simulink model "example_of_spead_control"  (R2021a)
settings: Solver=VariableStepAuto  StartTime=0.0  StopTime=10.0  RelTol=1e-3
libraries: simulink x1
settings Model: Creator=YasserNet  LastModifiedBy=YasserNet

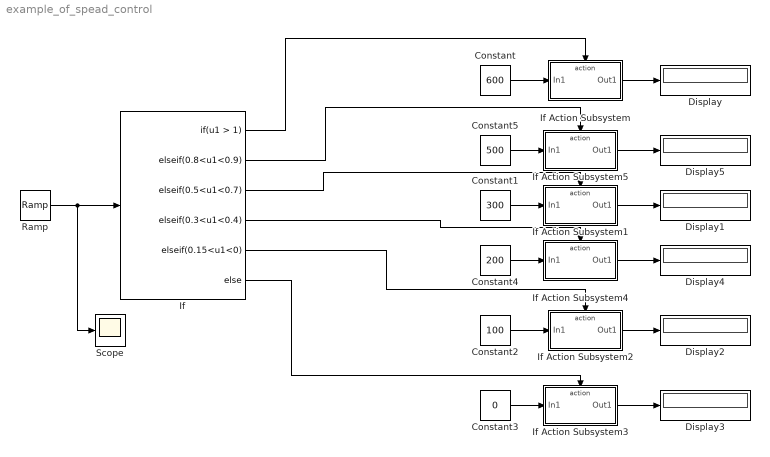
== system example_of_spead_control ==
  Constant : Constant  Value=600
  Constant1 : Constant  Value=300
  Constant2 : Constant  Value=100
  Constant3 : Constant  Value=0
  Constant4 : Constant  Value=200
  Constant5 : Constant  Value=500
  Display{,1..5} (6 alike) : Display
  If : If  IfExpression=u1 > 1  ElseIfExpressions=0.8<u1<0.9,0.5<u1<0.7,0.3<u1<0.4,0.15<u1<0
  If Action Subsystem : Subsystem  TreatAsAtomicUnit=on
  If Action Subsystem1 : Subsystem  TreatAsAtomicUnit=on
  If Action Subsystem2 : Subsystem  TreatAsAtomicUnit=on
  If Action Subsystem3 : Subsystem  TreatAsAtomicUnit=on
  If Action Subsystem4 : Subsystem  TreatAsAtomicUnit=on
  If Action Subsystem5 : Subsystem  TreatAsAtomicUnit=on
  Ramp : simulink/Sources/Ramp  slope=1  start=1  InitialOutput=6
  Scope : Scope
  wires:
  Ramp/1 -> Scope/1, If/1
  If Action Subsystem/1(Out1) -> Display/1
  Constant/1 -> If Action Subsystem/1(In1)
  Constant1/1 -> If Action Subsystem1/1(In1)
  If Action Subsystem1/1(Out1) -> Display1/1
  If Action Subsystem2/1(Out1) -> Display2/1
  Constant2/1 -> If Action Subsystem2/1(In1)
  Constant3/1 -> If Action Subsystem3/1(In1)
  If Action Subsystem3/1(Out1) -> Display3/1
  If Action Subsystem4/1(Out1) -> Display4/1
  Constant4/1 -> If Action Subsystem4/1(In1)
  Constant5/1 -> If Action Subsystem5/1(In1)
  If Action Subsystem5/1(Out1) -> Display5/1
  If/1 -> If Action Subsystem/Action
  If/2 -> If Action Subsystem5/Action
  If/6 -> If Action Subsystem3/Action
  If/3 -> If Action Subsystem1/Action
  If/4 -> If Action Subsystem4/Action
  If/5 -> If Action Subsystem2/Action

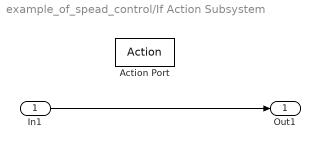
== system example_of_spead_control/If Action Subsystem ==
  In1 : Inport
  Action Port : ActionPort  ActionPortLabel=if(u1 > 1)
  Out1 : Outport
  wires:
  In1/1 -> Out1/1

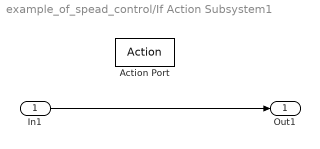
== system example_of_spead_control/If Action Subsystem1 ==
  In1 : Inport
  Action Port : ActionPort  ActionPortLabel=elseif(0.5<u1<0.7)
  Out1 : Outport
  wires:
  In1/1 -> Out1/1

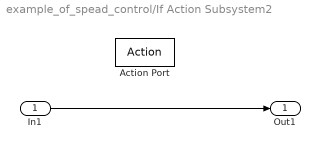
== system example_of_spead_control/If Action Subsystem2 ==
  In1 : Inport
  Action Port : ActionPort  ActionPortLabel=elseif(0.15<u1<0)
  Out1 : Outport
  wires:
  In1/1 -> Out1/1

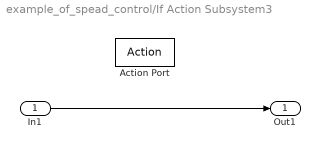
== system example_of_spead_control/If Action Subsystem3 ==
  In1 : Inport
  Action Port : ActionPort  ActionPortLabel=else
  Out1 : Outport
  wires:
  In1/1 -> Out1/1

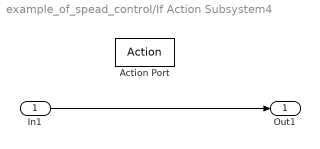
== system example_of_spead_control/If Action Subsystem4 ==
  In1 : Inport
  Action Port : ActionPort  ActionPortLabel=elseif(0.3<u1<0.4)
  Out1 : Outport
  wires:
  In1/1 -> Out1/1

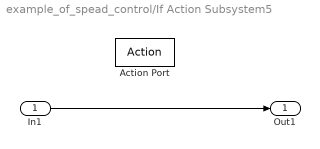
== system example_of_spead_control/If Action Subsystem5 ==
  In1 : Inport
  Action Port : ActionPort  ActionPortLabel=elseif(0.8<u1<0.9)
  Out1 : Outport
  wires:
  In1/1 -> Out1/1
